simulink model "hw3"  (R2020a)
settings: Solver=VariableStepAuto  StartTime=0.0  StopTime=1  RelTol=1e-3
undefined symbols (not defined in the file): Beq, D2R, Gr, Jeq, Ka_c, Ka_s, Kd_p, Ke, Ki_c, Ki_s, Kp_c, Kp_p, Kp_s, Kt, La, Ra
(part 2 of 2)

== system hw3/Subsystem9/Speed_Controller2 ==
  Load_Speed_ref : Inport
  Load_Speed_measurement : Inport  Port=2
  Add : Sum
  Integrator : Integrator
  Ka_s : Gain  Gain=Ka_s
  Ki_s : Gain  Gain=Ki_s
  Kp_s : Gain  Gain=Kp_s
  Saturation : Saturate  UpperLimit=27.3  LowerLimit=-27.3
  Sum : Sum  Inputs=|+-
  Sum1 : Sum  Inputs=-+|
  Sum2 : Sum  Inputs=|-+
  Current_ref : Outport  VectorParamsAs1DForOutWhenUnconnected=off
  wires:
  Integrator/1 -> Add/1
  Sum1/1 -> Ki_s/1
  Ki_s/1 -> Integrator/1
  Saturation/1 -> Sum2/1, Current_ref/1
  Load_Speed_measurement/1 -> Sum/2
  Ka_s/1 -> Sum1/1
  Sum2/1 -> Ka_s/1
  Add/1 -> Saturation/1, Sum2/2
  Load_Speed_ref/1 -> Sum/1
  Kp_s/1 -> Add/2
  Sum/1 -> Sum1/2, Kp_s/1
